simulink model "10_MCU_PMSM1_Trajectoire_dsPIC33CK_LVMC"  (R2023b)
settings: Solver=FixedStepDiscrete  StartTime=0.0  StopTime=10.0  FixedStep=5e-5  RelTol=1e-3  EnableMultiTasking=on
InitFcn:
  | %% Trajectoire Source
  | 
  | t0 = 0;
  | t1 = t0+0.1;
  | t2 = t1+0.1;
  | t3 = t2+0.5;
  | t4 = t3+0.2;
  | t5 = t4+0.5;
  | t6 = t5+0.2;
  | t7 = t6+0.1;
  | 
  | 
  | 
  | x = [t0 t1 t2 t3 t4 t5 t6 t7];
  | y = [0 0 0.25 0.25 1 1 0 0];
  | 
  | 
  | %% Trajectoire charge
  | t0 = 0;
  | t1 = t0+0.4;
  | t2 = t1+1e-2;
  | t3 = t2+0.1;
  | t4 = t3+1e-2;
  | t5 = 1.1;
  | t6 = t5+1e-2;
  | t7 = t6+0.1
  | t8 = t7+1e-2
  | t9 = 1.7;
  | x2 = [t0 t1 t2 t3 t4 t5 t6 t7 t8 t9];
  | y2 = [0 0 1 1 0 0 1 1 0 0];
undefined symbols (not defined in the file or in its folder): A0, A4, AN0, AN1, B0, B2, Bias1, Bias2, C12, C13, C14, C7, control, D11, D12, D13, D14, D5, D6, D7, diff, DiscIntNeverNeededParam, inverter, Max, MaxPer, model, ms, NumBits1, NumBits2, P20, P32, P55, P60, P61, P62, P69, P70, P71, P75, P76, P77, P78, Pin, pmsm, PosRange1, PosRange2, PWM1max, Resol, s, Slope1, Slope2, us
libraries: simulink x55, MCHP_Blockset x26
(part 1 of 4)
Description:
  | Speed vector control example
  | 
  | This example provides classical vector speed control
  | 
  | For mode details on the control strategy visit ctrl-elec.fr
  | 
  | Contacts :
  | Romain Delpoux (romain.delpoux@insa-lyon.fr)
  | Lubin Kerhuel (lubin.kerhuel@microchip.com)
settings Model: Creator=rdelpoux  LastModifiedBy=rdelpoux
settings OptimizationCC: DefaultParameterBehavior=Inlined  DefaultUnderspecifiedDataType=single  EnhancedBackFolding=on  BooleansAsBitfields=on  PassReuseOutputArgsAs=Individual arguments  ZeroExternalMemoryAtStartup=off  ZeroInternalMemoryAtStartup=off  OptimizeBlockOrder=speed  DifferentSizesBufferReuse=on  EfficientTunableParamExpr=on
settings DebuggingCC: MultiTaskCondExecSysMsg=none  ParameterTunabilityLossMsg=error
settings HardwareCC: ProdBitPerInt=16  ProdBitPerPointer=16  ProdBitPerSizeT=16  ProdBitPerPtrDiffT=32  ProdLargestAtomicInteger=Integer  ProdLargestAtomicFloat=None  ProdWordSize=16  ProdHWDeviceType=Generic->Custom
settings ModelReferenceCC: ModelReferenceNumInstancesAllowed=Single
settings SFSimCC: MATLABDynamicMemAlloc=off
settings RTWCC: Description=Microchip Embedded Target PIC24 dsPIC30 dsPIC33 (real-time)  SystemTargetFile=MCHP_dsPIC_stf.tlc  TemplateMakefile=MCHP_dsPIC.tmf
settings CodeAppCC: ForceParamTrailComments=on  IgnoreCustomStorageClasses=off  MaxIdLength=255  OperatorAnnotations=on  SimulinkDataObjDesc=on  SFDataObjDesc=on  InsertBlockDesc=on
settings STFCustomTargetCC: TargetLibSuffix=_lib.a  TargetLangStandard=C89/C90 (ANSI)  CodeReplacementLibrary=Microchip Code Replacement Library for dsPIC  MultiwordLength=256  CombineOutputUpdateFcns=on  CombineSignalStateStructs=on  SuppressErrorStatus=on  ERTCustomFileBanners=on  SupportContinuousTime=off  RemoveResetFunc=on  MATLABClassNameForMDSCustomization=Simulink.SoftwareTarget.ERTCustomization  SystemTargetFile=MCHP_dsPIC_stf.tlc
settings ERTTargetCC: TargetLibSuffix=_lib.a  CodeReplacementLibrary=Microchip Code Replacement Library for dsPIC  ParMdlRefBuildCompliant=off  CompOptLevelCompliant=off  ConcurrentExecutionCompliant=off  CombineSignalStateStructs=on  SuppressErrorStatus=on  SupportNonInlinedSFcns=on  ModelStepFunctionPrototypeControlCompliant=off  CPPClassGenCompliant=off  UseToolchainInfoCompliant=off  ExtModeStaticAllocSize=500  InlinedParameterPlacement=NonHierarchical  ERTSrcFileBannerTemplate=MCHP_dsPIC_code_template.cgt  ERTHdrFileBannerTemplate=MCHP_dsPIC_code_template.cgt  ERTDataSrcFileTemplate=MCHP_dsPIC_code_template.cgt  ERTDataHdrFileTemplate=MCHP_dsPIC_code_template.cgt  ERTCustomFileTemplate=MCHP_main.tlc  MaxLineWidth=110

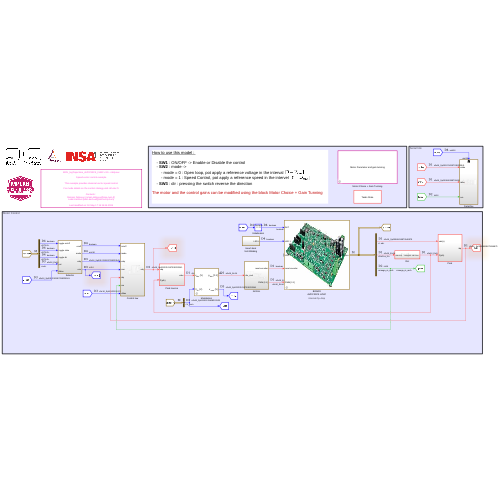
[thumbnail: Simulink's stored preview of the top-level diagram]
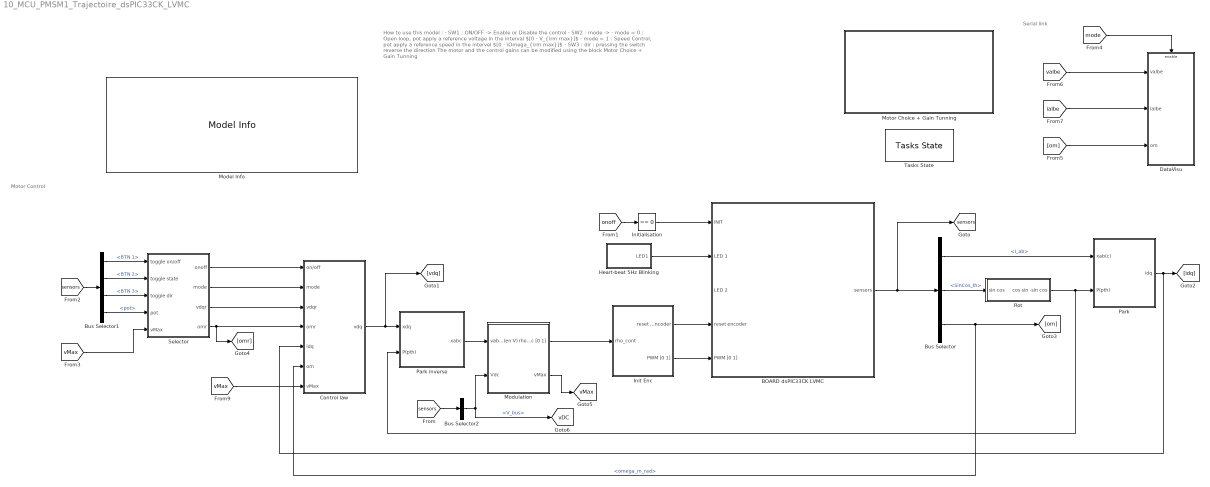
== system 10_MCU_PMSM1_Trajectoire_dsPIC33CK_LVMC ==
  note: How to use this model :
      |
      | - SW1 : ON/OFF -> Enable or Disable the control
      | - SW2 : mode ->
      | - mode = 0 : Open loop, pot apply a reference voltage in the interval $[0 - V_{\rm max}]$
      | - mode = 1 : Speed Control, pot apply a reference speed in the intervel $[0 - \Omega_{\rm max}]$
      | - SW3 : dir : pressing the switch reverse the direction
      |
      | The motor and the control gains can be modified using the block Motor Choice + Gain Tunning
  note: Motor Control
  note: Serial link
  BOARD dsPIC33CK LVMC : Subsystem  mask(dsPIC33CK Low Voltage Motor Control Board (LVMC) - dsPIC33CK256MP508){boardVariants=internal Op-Amp, n=model.p, QEIResolution=4*model.enclines, QEI_Reset=on logical input (software), QEI_Offset_settings=0, QEIOffset=0}
      mask prompts: boardVariants "board variants"; n "Motor poles pairs"; QEIResolution "Optical encoder resolution per mechanical rotation (lines)"; QEI_Reset "Optical encoder reset"; QEI_Offset_settings "Optical encoder offset (mechanical in rad)"; QEIOffset "Optical encoder offset (mechanical in rad)"
      mask help:
      | Template for motor control algorithm. Open subsystem (ctrl-u) for further customisation.
      |
      | Block bus output provices:
      |   - Current phase ia & ib, DC bus and potentiometer position
      |   - Buttons (0 when pressed)
      |   - QEI position and velocity
      |   - MCU load and overload
      |
      | Block inputs:
      |   - INIT signal average the current phase ia and ib to be removed
      |   - LEDs
      |   - Reset encoder allows to align the motor while reseting the encoder
      |   - PWM normalized duty cycle value
      |
      | Model 50us base rate (20kHz) is synchronized with ADC conversion which is synchronized with the 50us PWM periods
      mask init:
      | BlksQEI = find_system(gcb,'FollowLinks','on','LookUnderMasks','all','ReferenceBlock','MCHP_Blockset/QEI/QEI');
      | QEI_Reset = get_param(gcb,'QEI_Reset');
      | if numel(BlksQEI) >= 1
      |     switch QEI_Reset
      |         case 'on index signal'
      |             set_param(BlksQEI{1},'PIMOD_mode','RESET position on each INDEX event');
      |         case 'on logical input (software)'        
      |             set_param(BlksQEI{1},'PIMOD_mode','position is cyclique between user defined boundaries'); 
      |         case 'custom setting'
      |             % do nothing 
      |     end
      | end % if
      | 
      | 
      |     BlksOpAmp = find_system(gcb,'FollowLinks','on','IncludeCommented','on','LookUnderMasks','all','ReferenceBlock','MCHP_Blockset/Analog IO/Op-Amp');
      |     if numel(BlksOpAmp) >= 1
      |         boardVariants = get_param(gcb,'boardVariants');
      |         switch boardVariants
      |             case 'internal Op-Amp'
      |                 set_param(BlksOpAmp{1},'Commented','off');
      |             case 'external Op-Amp'
      |                 set_param(BlksOpAmp{1},'Commented','on');
      |         end
      |     end % if
      settings: AttributesFormatString=%<boardVariants>
      mask TypeOptions boardVariants: internal Op-Amp | external Op-Amp
      mask TypeOptions QEI_Reset: on index signal | on logical input (software) | custom setting
      mask Callback QEI_Reset:
      | QEI_Reset = get_param(gcb,'QEI_Reset');
      | switch QEI_Reset
      |     case 'on index signal'
      |         QEIOffset = MCHP_Fun.Evalin('base','QEIOffset');
      |         set_param(gcb,'QEIOffset',num2str(QEIOffset));
      |         set_param(gcb,'MaskVisibilities',{'on';'on';'on';'on';'on';'off'});
      |     case 'on logical input (software)'
      |         set_param(gcb,'QEIOffset','0');
      |         set_param(gcb,'MaskVisibilities',{'on';'on';'on';'on';'off';'off'});
      |     case 'custom setting'
      |         set_param(gcb,'MaskVisibilities',{'on';'on';'on';'on';'on';'off'});
      |         % do nothing
      | end
      mask DialogControl boardVariants Tooltip: Default board use internal Op-Amp
      mask DialogControl n Tooltip: Number of pole pairs of the motor
      mask DialogControl QEIResolution Tooltip: encoder resolution per mechanical rotation
      mask DialogControl QEI_Reset Tooltip: enable encoder index signal if available. Otherwise align motor by applying a tension and set the rst input to 1
      mask DialogControl QEI_Offset_settings Tooltip: offset angle between encoder index and motor winding reference axis applied on theta_m and theta_e
      mask Display: image('MCHP_i_Board_LVMC_reduced.jpg');
  Bus Selector : BusSelector  OutputSignals=ADC.I_ab,optical coder.elec.SinCos_th,optical coder.mecc.omega_m_rad
  Bus Selector1 : BusSelector  OutputSignals=BTN.BTN 1,BTN.BTN 2,BTN.BTN 3,ADC.pot
  Bus Selector2 : BusSelector  OutputSignals=ADC.V_bus
  Control law : Subsystem
      settings: LibrarySourceBlock=insa_control_base/Control law
  DataVisu : Subsystem
  Heart-beat 5Hz Blinking : Subsystem
  Init Enc : Subsystem
  Initialisation : simulink/Logic and Bit Operations/Compare To Constant  relop===  const=0  OutDataTypeStr=boolean
  Model Info : simulink/Model-Wide Utilities/Model Info  Frame=on  DisplayStringWithTags=|  HorizontalTextAlignment=Center  LeftAlignmentValue=0.5
      | %<ModelName> v%<ModelVersion> - %<Creator>
      | 
      | %<Description>
      | 
      | Last modified on: %<LastModificationDate>
  Modulation : Subsystem  mask{modulation=Space Vector, mod=0}
      mask init:
      | switch modulation
      |     case 'Sinusoidale'
      |         mod = 0;
      |     otherwise
      |         mod = 1;
      | end
      mask TypeOptions modulation: Sinusoidale | Space Vector
      mask DialogControl DescGroupVar Prompt: Modulation interssecticve
      mask DialogControl DescTextVar Prompt: Choose between sinus or space vector modulation
      mask Display:
      | port_label('output', 1, '\rho_{abc} [0 1]', 'texmode','on')
      | port_label('output', 2, 'v_{\rm max} (V)', 'texmode','on')
      | port_label('input', 1, 'v_{abc} (V)', 'texmode','on')
      | port_label('input', 2, 'V_{dc} (V)', 'texmode','on')
  Motor Choice + Gain Tunning : Subsystem  mask(INSA motor control gain tunning){presetMotor=Teknic-2310P, modelPMSM=Teknic-2310P, p=4, R=0.656, L=0.00035, Phif=0.0066, J=1e-05, F=1e-05, C0=0.01, vMax=48, iMax=10, omegaMax=500, enclines=1000, zetaE=0.7, trE=3*model.L/model.R, trWnE=3, KpE=0.2624, KiE=-1229.5314, zetaM=1.0, trM=0.05, trWnM=5, KpM=0.050253, KiM=-2.5253, tsMeca=1e-3}
      mask prompts: presetMotor "Predefined motor"; modelPMSM "PMSM model"; p "Poles pairs p"; R "Phase resistor R (Ohm)"; L "Phase inductance L (H)"; Phif "Flux constant Phif (Wb)"; J "Intertia J (kg.m^2)"; F "Damping coefficient F (N.m.s/rad)"; C0 "Coulomb friction C0 (N.m)"; vMax "Max Voltage (V)"; iMax "Max Current iMax (A)"; omegaMax "Max Speed (rad/s)"; enclines "Lines (RAW)"; zetaE "Damping factor (zeta)"; trE "Time response (s)"; trWnE "TrWn (3 for zeta = 0.7)"; KpE "Kp"; KiE "Ki"; zetaM "Damping factor (zeta)"; trM "Time response (s)"; trWnM "TrWn (3 for zeta = 0.7)"; KpM "Kp"; KiM "Ki"; tsMeca "Mecanical Sampling Time (s)"
      mask help: The bloc provides basic gain tunning solution based on pole placement.
      mask init:
      | % Mototor definition
      | model = struct;
      |          
      | switch presetMotor
      |     case 'Teknic-2310P'
      |         model.modelPMSM    = 'Teknic-2310P';                                 %           // Manufacturer Model Number
      |         model.p        = 4;                                                  %           // Pole Pairs for the motor
      |         model.R        = 0.656;                                              %Ohm        // Stator Resistor
      |         model.L        = 0.35e-3;                                            %H          // Inductance value
      |         model.Phif     = 6.6e-3;                                             %Wb         // PM flux
      |         model.J        = 1e-05;                                              %Kg-m2      // Inertia in SI units
      |         model.F        = 1.e-05;                                             %Kg-m2/s    // Friction Co-efficient
      |         model.C0       = 0.01;                                               %Kg-m2      // Dry friction
      |         model.vMax     = 48;                                                 %V          // Max voltage      
      |         model.iMax     = 10;                                                 %A          // Max current
      |         model.omegaMax = 500;                                                %rad/spm    // Max speed
      |         model.enclines = 1000;                                               % top       // Encoder top per round
      |     case 'Short HURST (AC300020)'
      |         model.modelPMSM    = 'Short HURST (AC300020)';                       %           // Manufacturer Model Number
      |         model.p        = 5;                                                  %           // Pole Pairs for the motor
      |         model.R        = 2.015;                                              %Ohm        // Stator Resistor
      |         model.L        = 2.3e-3;                                             %H          // Inductance value
      |         model.Phif     = 3.3e-3;                                             %Wb         // PM flux
      |         model.J        = 1.908e-04;                                          %Kg-m2      // Inertia in SI units
      |         model.F        = 1.044e-04;                                          %Kg-m2/s    // Friction Co-efficient
      |         model.C0       = 0.01;                                               %Kg-m2      // Dry friction
      |         model.vMax     = 48;                                                 %V          // Max voltage      
      |         model.iMax     = 10;                                                 %A          // Max current
      |         model.omegaMax = 350;                                                %rad/spm    // Max speed    
      |         model.enclines = NaN;                                                % top       // Encoder top per round
      |     case 'Long HURST (AC300022)'
      |         model.modelPMSM    = 'Long HURST (AC300022)';                        %           // Manufacturer Model Number
      |         model.p        = 5;                                                  %           // Pole Pairs for the motor
      |         model.R        = 0.405;                                              %Ohm        // Stator Resistor
      |         model.L        = 0.30e-3;                                            %H          // Inductance value
      |         model.Phif     = 7.63e-3;                                            %Wb         // PM flux
      |         model.J        = 1.908e-04;                                          %Kg-m2      // Inertia in SI units
      |         model.F        = 1.044e-04;                                          %Kg-m2/s    // Friction Co-efficient
      |         model.C0       = 0.01;                                               %Kg-m2      // Dry friction
      |         model.vMax     = 48;                                                 %V          // Max voltage      
      |         model.iMax     = 10;                                                 %A          // Max current
      |         model.omegaMax = 350;                                                %rad/spm    // Max speed    
      |         model.enclines = 250;                                                % top       // Encoder top per round
      |     case 'Custom'
      |         model.modelPMSM    = 'Custom';                                       %           // Manufacturer Model Number
      |         model.p        = p;                                                  %           // Pole Pairs for the motor
      |         model.R        = R;                                                  %Ohm        // Stator Resistor
      |         model.L        = L;                                                  %H          // Inductance value
      |         model.Phif     = Phif;                                               %Wb         // PM flux
      |         model.J        = J;                                                  %Kg-m2      // Inertia in SI units
      |         model.F        = F;                                                  %Kg-m2/s    // Friction Co-efficient
      |         model.C0       = C0;                                                 %Kg-m2      // Dry friction
      |         model.vMax     = vMax;                                               %V          // Max voltage      
      |         model.iMax     = iMax;                                               %A          // Max current
      |         model.omegaMax = omegaMax;                                           %rad/spm    // Max speed
      |         model.enclines = enclines;                                           % top       // Encoder top per round
      | end
      | 
      | 
      | 
      | ff = fields(model);
      | for i=1:numel(ff)
      |     set_param(gcb,ff{i},num2str(model.(ff{i})) );
      | end
      | %% Define fracation length for fixed point datatype
      | model.FracLen.curr  = (15-ceil(log2(model.iMax)));  % Fraction length for current variables
      | model.FracLen.volt  = (15-ceil(log2(model.vMax)));    % Fraction length for voltage variables
      | model.FracLen.volt2 = (15-ceil(log2(2*model.vMax^2))); % Fraction length for voltage square variables
      | model.FracLen.invsqrtvolt = (15-ceil(log2(1/sqrt(model.vMax/4)^2))); % Fraction length for voltage square variables
      | 
      | 
      | %% LUT 1/sqrt(||v_dq||)
      | func = '1./sqrt(x)';
      | xmin = (model.vMax/4)^2; xmax = 2*model.vMax^2;
      | 
      | xdt = sfix(16); xscale = 2^-(15-ceil(log2(xmax)));
      | ydt = sfix(16); yscale = 2^-(15-ceil(log2(1./sqrt(xmin))));
      | rndmeth = 'Floor';
      | errmax = [];
      | nptsmax = [128];
      | spacing = 'even';
      | 
      | %Compute LUT
      | [model.math.LUTintsqrtx,model.math.LUTintsqrty] = fixpt_look1_func_approx(func,xmin,xmax,xdt,xscale,ydt,yscale,rndmeth,errmax,nptsmax,spacing);
      | 
      | 
      | assignin('base','model',model);
      | 
      | %% Define control structure 
      | control = struct;
      | control.tauElec = model.L/model.R;
      | control.kElec = 1/model.R;
      | control.tauMeca = model.J/model.F;
      | control.kMeca = 3/2*model.p*model.Phif/model.F;
      | 
      | 
      | control.trDElec = trE;
      | control.zetaDElec = zetaE;
      | control.trwnDElec = trWnE;
      | control.wnDElec = control.trwnDElec/control.trDElec;
      | control.kE = [(2*control.zetaDElec*control.wnDElec*control.tauElec-1)/control.kElec, ...
      |                 -control.tauElec*control.wnDElec^2/control.kElec];
      | set_param(gcb, 'KpE', num2str(control.kE(1)));
      | set_param(gcb, 'KiE', num2str(control.kE(2)));
      | 
      | control.trDMeca = trM;
      | control.zetaDMeca = zetaM;
      | control.trwnDMeca = trWnM;
      | control.wnDMeca = control.trwnDMeca/control.trDMeca;
      | control.kM = [(2*control.zetaDMeca*control.wnDMeca*control.tauMeca-1)/control.kMeca, ...
      |                 -control.tauMeca*control.wnDMeca^2/control.kMeca];
      | set_param(gcb, 'KpM', num2str(control.kM(1)));
      | set_param(gcb, 'KiM', num2str(control.kM(2)));
      | 
      | control.tsMeca = tsMeca;
      | 
      | assignin('base','control',control);
      mask Help: For more help on the gain tunning, visit http://rcp.ctrl-elec.fr
      mask TypeOptions presetMotor: Custom | Teknic-2310P | Short HURST (AC300020) | Long HURST (AC300022)
      mask DialogControl DescGroupVar Prompt: Moteur Synchrone à aimants permanents
      mask DialogControl DescTextVar Prompt: Motor Parameters for gain tunning
      mask DialogControl Container4 Prompt: Motor Parameters
      mask DialogControl Container7 Prompt: Parameters
      mask DialogControl Container8 Prompt: Electrical parameters
      mask DialogControl Container9 Prompt: Mechanical parameters
      mask DialogControl Container13 Prompt: Motor Limits
      mask DialogControl Container14 Prompt: Encoder
      mask DialogControl Container10 Prompt: Gain Tuning
      mask DialogControl Control2 Prompt: Pole placement
      mask DialogControl Container11 Prompt: Electrical Dynamic
      mask DialogControl Container12 Prompt: Mechanical Dynamic
      mask Display: disp('Motor Parameter and gain tunning');
  Park : Subsystem
  Park inverse : Subsystem
  Rot : Subsystem
  Selector : Subsystem
  Tasks State : MCHP_Blockset/Profiling/Tasks State  TasksPin=E0 D2 D9 C8  MCHP_PORT={Task D1 Running}{Task D1}15:1:E0;{Task D2 Running}{Task D2}15:1:D2;{Task D3 Running}{Task D3}15:1:D9;{Task D4 Running}{Task D4}15:1:C8;  MCHP_MASTERLINK=MCU_logTrajectoire_dsPIC33CK_LVMC/BOARD dsPIC33CK LVMC/Microchip Master
      settings: SourceProductName=MPLAB Device Blocks for Simulink
  tag scope: sensors=global, vDC=global, vMax=global
  wires:
  Rot/1("cos sin -sin cos ") -> Park/2(P(pth)), Park inverse/2(P(pth))
  Init Enc/1(reset encoder) -> BOARD dsPIC33CK LVMC/4(reset encoder)
  Init Enc/2(PWM [0 1]) -> BOARD dsPIC33CK LVMC/5(PWM [0 1])
  Park inverse/1(xabc) -> Modulation/1("vabc (en V) ")
  Park/1(idq) -> Control law/5(idq), [idq]
  [vMax] -> Selector/5(vMax)
  Modulation/2(vMax) -> [vMax]
  [vMax] -> Control law/7(vMax)
  Selector/1(onoff) -> Control law/1(on/off)
  [om] -> DataVisu/3(om)
  Selector/4(omr) -> Control law/4(omr), [omr]
  Bus Selector/3 -> Control law/6(om), [om]  "<omega_m_rad>"
  [valbe] -> DataVisu/1(valbe)
  [ialbe] -> DataVisu/2(ialbe)
  Bus Selector2/1 -> Modulation/2(Vdc), [vDC]  "<V_bus>"
  [sensors] -> Bus Selector2/1
  Selector/2(mode) -> Control law/2(mode)
  Selector/3(vdqr) -> Control law/3(vdqr)
  [sensors] -> Bus Selector1/1
  Control law/1(vdq) -> Park inverse/1(xdq), [vdq]
  Bus Selector/2 -> Rot/1(sin cos)  "<SinCos_th>"
  Bus Selector/1 -> Park/1(xab(c))  "<I_ab>"
  BOARD dsPIC33CK LVMC/1(sensors) -> [sensors], Bus Selector/1
  Heart-beat 5Hz Blinking/1(LED1) -> BOARD dsPIC33CK LVMC/2(LED 1)
  [onoff] -> Initialisation/1
  Initialisation/1 -> BOARD dsPIC33CK LVMC/1(INIT)
  Modulation/1(rho_abc [0 1]) -> Init Enc/1(rho_cont)
  Bus Selector1/1 -> Selector/1(toggle on/off)  "<BTN 1>"
  Bus Selector1/2 -> Selector/2(toggle state)  "<BTN 2>"
  Bus Selector1/3 -> Selector/3(toggle dir)  "<BTN 3>"
  Bus Selector1/4 -> Selector/4(pot)  "<pot>"
  [mode] -> DataVisu/Enable
